simulink model "E0422_servo"  (R2024b)
settings: Solver=VariableStepAuto  StartTime=0.0  StopTime=10.0  RelTol=1e-3
values from neighbouring files (symbols this model uses):
  K = 1.91    [Ejemplo0409_lgr.m]    (also in Ejemplo0422_KhK.m = 0.156; Ejemplo0506_compensadoradelanto.m = 11; Ejemplo0508_retraso.m = 0.80:0.01:1.1; Ejemplo0527_criterionyquist.m = 1)
  Kh = 0.c    [Ejemplo0422_KhK.m]
settings Model: Creator=carlosjuarez  LastModifiedBy=carlosjuarez

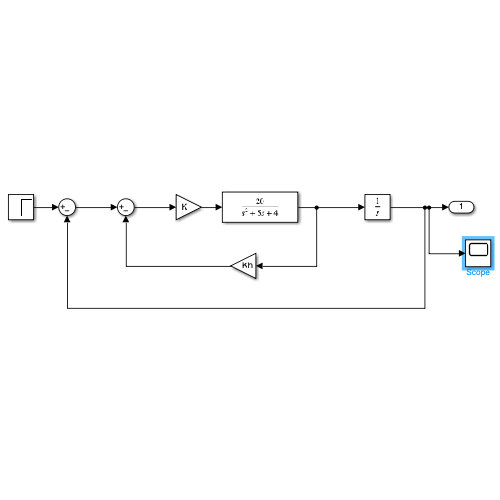
[thumbnail: Simulink's stored preview of the top-level diagram]
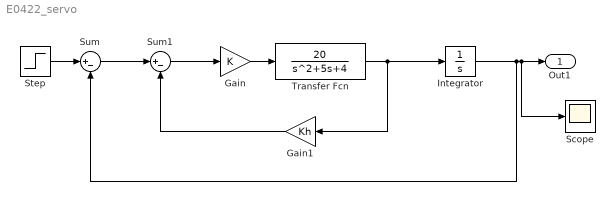
== system E0422_servo ==
  Gain : Gain  Gain=K
  Gain1 : Gain  Gain=Kh
  Integrator : Integrator
  Scope : Scope
  Step : Step  SampleTime=0
  Sum : Sum  Inputs=|+-
  Sum1 : Sum  Inputs=|+-
  Transfer Fcn : TransferFcn  Numerator=[20]  Denominator=[1,5,4]
  Out1 : Outport
  wires:
  Sum1/1 -> Gain/1
  Gain/1 -> Transfer Fcn/1
  Transfer Fcn/1 -> Gain1/1, Integrator/1
  Sum/1 -> Sum1/1
  Step/1 -> Sum/1
  Integrator/1 -> Sum/2, Scope/1, Out1/1
  Gain1/1 -> Sum1/2
